simulink model "generalModelForErrorsNEW"  (R2016b)
settings: Solver=ode15s  StartTime=0  StopTime=3500  FixedStep=0.0001  MaxStep=0.001  RelTol=1e-3
values from neighbouring files (symbols this model uses):
  bigpump_const = 1    [run_model.m]
  gain_coef = 4000*10    (= 40000)    [params.m]    (also in run_model.m)
  min_vol = 20    [params.m]
  minipump_const = 0    [run_model.m]
  pipe_diameter = 2    [params.m]
  pressurization = 100000    [params.m]
  pump_speed = 20000    [params.m]
  valve_gain = 0.01    [params.m]
  ws_fault_time = fault_time    [run_model.m]
  ws_sample_time_end_valve_bigpump_in = 0    [run_model.m]
  ws_sample_time_end_valve_bigpump_out = 0    [run_model.m]
  ws_sample_time_end_valve_car_tank = 0    [run_model.m]
  ws_sample_time_end_valve_cartank1_in = 0    [run_model.m]
  ws_sample_time_end_valve_cartank1_out = 0    [run_model.m]
  ws_sample_time_end_valve_cartank2_in = 0    [run_model.m]
  ws_sample_time_end_valve_cartank2_out = 0    [run_model.m]
  ws_sample_time_end_valve_cartank3_in = 0    [run_model.m]
  ws_sample_time_end_valve_cartank3_out = 0    [run_model.m]
  ws_sample_time_end_valve_general_tank = 0    [run_model.m]
  ws_sample_time_end_valve_minipump_in = 0    [run_model.m]
  ws_sample_time_end_valve_minipump_out = 0    [run_model.m]
undefined symbols (not defined in the file or in its folder): sigbuilder_block
libraries: sh_lib x61, nesl_utility x34, fl_lib x32, powerlib_meascontrol x2
(part 1 of 2)
settings Model: Creator=plotb  LastModifiedBy=plotb
settings SimscapeCC: SimscapeLogDataHistory=10000

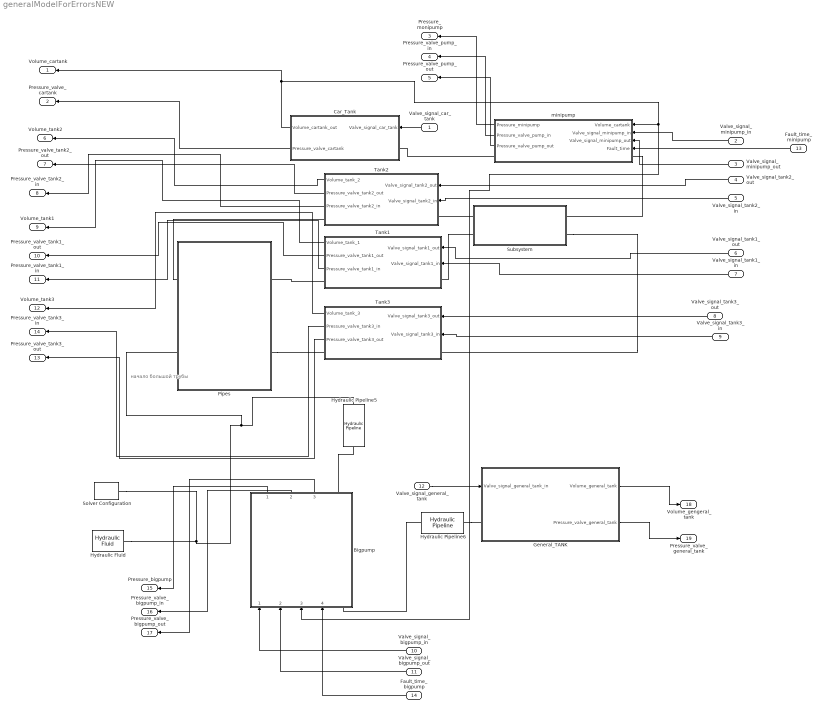
== system generalModelForErrorsNEW ==
  note: начало большой трубы
  Valve_signal_car_tank : Inport
  Valve_signal_minipump_in : Inport  Port=2
  Valve_signal_minipump_out : Inport  Port=3
  Valve_signal_tank2_out : Inport  Port=4
  Valve_signal_tank2_in : Inport  Port=5
  Valve_signal_tank1_out : Inport  Port=6
  Valve_signal_tank1_in : Inport  Port=7
  Valve_signal_tank3_out : Inport  Port=8
  Valve_signal_tank3_in : Inport  Port=9
  Valve_signal_bigpump_in : Inport  Port=10
  Valve_signal_bigpump_out : Inport  Port=11
  Valve_signal_general_tank : Inport  Port=12
  Fault_time_minipump : Inport  Port=13
  Fault_time_bigpump : Inport  Port=14
  Bigpump : Subsystem
  Car_Tank : Subsystem
  General_TANK : Subsystem
  Hydraulic Fluid : sh_lib/Hydraulic Utilities/Hydraulic Fluid  DataSource=1  SelFluid=21  SysTemp=temp  TrapAir=0.005  ViscDerFactor=1  range_error=1
  Hydraulic Pipeline5 : sh_lib/Pipelines/Hydraulic Pipeline  cs_type=1  d_in=pipe_diameter*2 m  area=1e-4 m^2  D_h=0.0112 m  s_factor=64  length=pipe_length_long m  length_ad=1 m  roughness=1.5e-5 m  Re_lam=2e+3  Re_turb=4e+3  wall_type=1  pr_r_coef=2e-12 m/Pa  time_const=0.01 s  k_sh=1.4  initial_pressure=initial_pressure Pa
  Hydraulic Pipeline6 : sh_lib/Pipelines/Hydraulic Pipeline  cs_type=1  d_in=pipe_diameter*2 m  area=1e-4 m^2  D_h=0.0112 m  s_factor=64  length=pipe_length_long m  length_ad=1 m  roughness=1.5e-5 m  Re_lam=2e+3  Re_turb=4e+3  wall_type=1  pr_r_coef=2e-12 m/Pa  time_const=0.01 s  k_sh=1.4  initial_pressure=initial_pressure Pa
  Pipes : Subsystem
  Solver Configuration : nesl_utility/Solver Configuration  PhysicalDomain=network_engine_domain  SubClassName=solver  LeftPortType=input  RightPortType=generic  Accelerate=off  Tones=[]  Harmonics=[]  SimulateNoise=off  Profile=off  UseLocalSampling=off  EnableSwitchedLinearOptims=on  FrequencyDomain=off  UseCCode=off  RelTol=0.001  AbsTol=1e-06  MinStep=1e-09  ToWorkspace=off  RevertToSquareIcSolve=off  NumHomotopyIterations=100  PhasorMode=off  PhasorModeNumHarmonics=1  OverrideAbsTol=off  DoDC=off  ResidualTolerance=1e-09  UseLocalSolver=off  LocalSolverChoice=NE_BACKWARD_EULER_ADVANCER  LocalSolverSampleTime=0.001  DoFixedCost=off  MaxNonlinIter=3  MaxModeIter=2  LinearAlgebra=Sparse  DelaysMemoryBudget=1024  AutomaticFiltering=on  FilteringTimeConstant=0.001
  Subsystem : Subsystem
  Tank1 : Subsystem
  Tank2 : Subsystem
  Tank3 : Subsystem
  minipump : Subsystem
  Volume_cartank : Outport
  Pressure_valve_cartank : Outport  Port=2
  Pressure_monipump : Outport  Port=3
  Pressure_valve_pump_in : Outport  Port=4
  Pressure_valve_pump_out : Outport  Port=5
  Volume_tank2 : Outport  Port=6
  Pressure_valve_tank2_out : Outport  Port=7
  Pressure_valve_tank2_in : Outport  Port=8
  Volume_tank1 : Outport  Port=9
  Pressure_valve_tank1_out : Outport  Port=10
  Pressure_valve_tank1_in : Outport  Port=11
  Volume_tank3 : Outport  Port=12
  Pressure_valve_tank3_out : Outport  Port=13
  Pressure_valve_tank3_in : Outport  Port=14
  Pressure_bigpump : Outport  Port=15
  Pressure_valve_bigpump_in : Outport  Port=16
  Pressure_valve_bigpump_out : Outport  Port=17
  Volume_gengeral_tank : Outport  Port=18
  Pressure_valve_general_tank : Outport  Port=19
  wires:
  Tank2/1(Volume_tank_2) -> Volume_tank2/1
  General_TANK/1(Volume_general_tank) -> Volume_gengeral_tank/1
  Tank1/1(Volume_tank_1) -> Volume_tank1/1
  Tank3/1(Volume_tank_3) -> Volume_tank3/1
  Valve_signal_car_tank/1 -> Car_Tank/1(Valve_signal_car_tank)
  Valve_signal_minipump_in/1 -> minipump/2(Valve_signal_minipump_in)
  Valve_signal_minipump_out/1 -> minipump/3(Valve_signal_minipump_out)
  Valve_signal_tank2_out/1 -> Tank2/1(Valve_signal_tank2_out)
  Valve_signal_tank2_in/1 -> Tank2/2(Valve_signal_tank2_in)
  Valve_signal_tank1_out/1 -> Tank1/1(Valve_signal_tank1_out)
  Valve_signal_tank1_in/1 -> Tank1/2(Valve_signal_tank1_in)
  Valve_signal_tank3_out/1 -> Tank3/1(Valve_signal_tank3_out)
  Valve_signal_tank3_in/1 -> Tank3/2(Valve_signal_tank3_in)
  Valve_signal_bigpump_in/1 -> Bigpump/1(Valve_signal_bigpump_in)
  Valve_signal_bigpump_out/1 -> Bigpump/2(Valve_signal_bigpump_out)
  Valve_signal_general_tank/1 -> General_TANK/1(Valve_signal_general_tank_in)
  Car_Tank/2(Pressure_valve_cartank) -> Pressure_valve_cartank/1
  Car_Tank/1(Volume_cartank_out) -> Bigpump/3(Volume_cartank), minipump/1(Volume_cartank), Volume_cartank/1
  Fault_time_minipump/1 -> minipump/4(Fault_time)
  minipump/1(Pressure_minipump) -> Pressure_monipump/1
  minipump/2(Pressure_valve_pump_in) -> Pressure_valve_pump_in/1
  minipump/3(Pressure_valve_pump_out) -> Pressure_valve_pump_out/1
  Tank2/2(Pressure_valve_tank2_out) -> Pressure_valve_tank2_out/1
  Tank2/3(Pressure_valve_tank2_in) -> Pressure_valve_tank2_in/1
  Tank1/2(Pressure_valve_tank1_out) -> Pressure_valve_tank1_out/1
  Tank1/3(Pressure_valve_tank1_in) -> Pressure_valve_tank1_in/1
  Tank3/2(Pressure_valve_tank3_in) -> Pressure_valve_tank3_in/1
  Tank3/3(Pressure_valve_tank3_out) -> Pressure_valve_tank3_out/1
  Fault_time_bigpump/1 -> Bigpump/4(Fault_time_bigpump)
  Bigpump/1(Pressure_bigpump) -> Pressure_bigpump/1
  Bigpump/2(Pressure_valve_bigpump_in) -> Pressure_valve_bigpump_in/1
  Bigpump/3(Pressure_valve_bigpump_out) -> Pressure_valve_bigpump_out/1
  General_TANK/2(Pressure_valve_general_tank) -> Pressure_valve_general_tank/1
  connections:
  minipump/LConn1 -- Subsystem/RConn1
  Subsystem/LConn1 -- Tank2/LConn1
  Subsystem/LConn2 -- Tank1/LConn1
  Hydraulic Fluid/RConn1 -- Pipes/LConn2 -- Hydraulic Pipeline5/LConn1 -- Solver Configuration/RConn1
  Tank2/RConn1 -- Pipes/LConn1
  Tank1/RConn1 -- Pipes/RConn1
  Pipes/RConn2 -- Tank3/RConn1
  Hydraulic Pipeline6/RConn1 -- General_TANK/LConn1
  Hydraulic Pipeline6/LConn1 -- Bigpump/LConn1
  Hydraulic Pipeline5/RConn1 -- Bigpump/RConn1
  minipump/RConn1 -- Car_Tank/LConn1
  Subsystem/RConn2 -- Tank3/LConn1

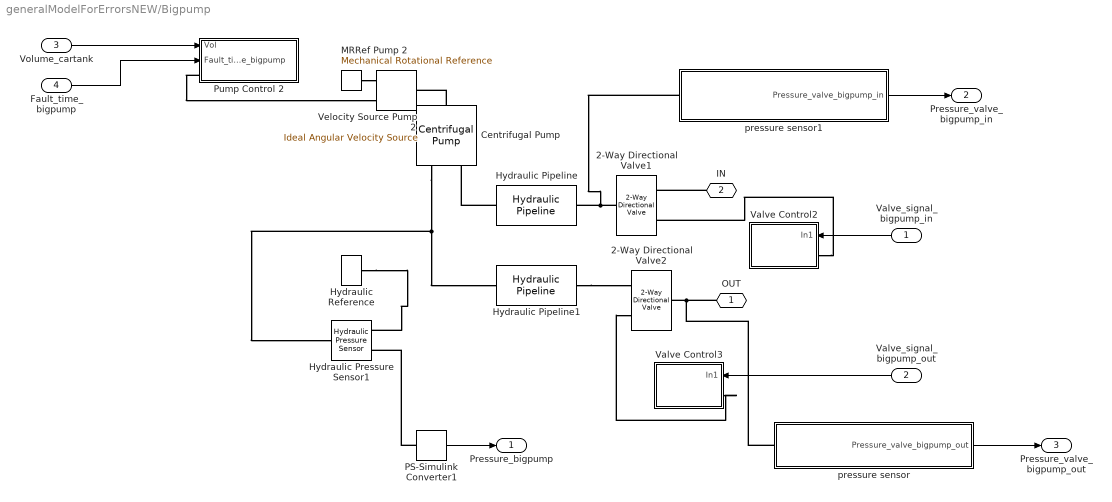
== system generalModelForErrorsNEW/Bigpump ==
  Valve_signal_bigpump_in : Inport
  Valve_signal_bigpump_out : Inport  Port=2
  Volume_cartank : Inport  Port=3
  Fault_time_bigpump : Inport  Port=4
  2-Way Directional Valve1 : sh_lib/Valves/Directional Valves/2-Way Directional Valve  mdl_type=1  area_max=passage_max_area_big_pipe m^2  opening_max=valve_stroke m  opening_tab=[ -0.002 0 0.002 0.005 0.015 ] m  area_tab=[ 1e-9 2.0352e-7 4.0736e-5 1.1438e-4 3.4356e-4 ] m^2  pressure_tab=[ -1e+7 -5e+6 -2e+6 2e+6 5e+6 1e+7 ] Pa  flow_rate_tab=[ -1e-7 -7.0711e-8 -4.4721e-8 4.4721e-8 7.0711e-8 1e-7; -2.0352e-5 -1.4391e-5 -9.1017e-6 9.1017e-6 1.4391e-5 2.0352e-5; -0.0040736 -0.0028805 -0.0018218 0.0018218 0.0028805 0.0040736; -0.011438 -0.0080879 -0.0051152 0.0051152 0.0080879 0.011438; -0.034356 -0.024293 -0.015364 0.015364 0.024293 0.034356 ] m^3/s  interp_method=1  extrap_method=1  C_d=0.7  x_0=valve_stroke m  Re_cr=12  A_leak=1e-12 m^2
  2-Way Directional Valve2 : sh_lib/Valves/Directional Valves/2-Way Directional Valve  mdl_type=1  area_max=passage_max_area_big_pipe m^2  opening_max=valve_stroke m  opening_tab=[ -0.002 0 0.002 0.005 0.015 ] m  area_tab=[ 1e-9 2.0352e-7 4.0736e-5 1.1438e-4 3.4356e-4 ] m^2  pressure_tab=[ -1e+7 -5e+6 -2e+6 2e+6 5e+6 1e+7 ] Pa  flow_rate_tab=[ -1e-7 -7.0711e-8 -4.4721e-8 4.4721e-8 7.0711e-8 1e-7; -2.0352e-5 -1.4391e-5 -9.1017e-6 9.1017e-6 1.4391e-5 2.0352e-5; -0.0040736 -0.0028805 -0.0018218 0.0018218 0.0028805 0.0040736; -0.011438 -0.0080879 -0.0051152 0.0051152 0.0080879 0.011438; -0.034356 -0.024293 -0.015364 0.015364 0.024293 0.034356 ] m^3/s  interp_method=1  extrap_method=1  C_d=0.7  x_0=valve_stroke m  Re_cr=12  A_leak=1e-12 m^2
  Centrifugal Pump : sh_lib/Pumps and Motors/Centrifugal Pump  mdl_type=1  c_1=326.8 Pa/(kg/m^3)  c_2=3.104e+4 Pa*s/kg  c_3=1.097e+7 Pa*s^2/(kg*m^3)  c_4=2.136e+5 Pa*s^2/(kg*m^3)  c_f=0.8  design_del=130 lpm  ref_velocity=1.77e+3 rpm  ref_density=920 kg/m^3  leak_resistance=1e+8 Pa/(m^3/s)  T_const=0.1 N*m  trq_press_coeff=1e-6 N*m/Pa  pump_del_1D=[ 0 28 90 130 154 182 ] lpm  press_diff_1D=[ 2.6 2.4 2 1.6 1.2 0.8 ] bar  pump_del_power_1D=[ 0 20 40 60 80 100 120 140 160 ] lpm  power_1D=[ 220 280 310 360 390 420 480 500 550 ] W  pump_del_2D=[ 0 50 100 150 200 250 300 350 ] lpm  pump_vel_2D=[ 3.2e+3 3.3e+3 3.4e+3 3.5e+3 ] rpm  press_diff_2D=[ 8.300000000000001 8.800000000000001 9.300000000000001 9.9; 7.8 8.300000000000001 8.800000000000001 9.4; 7.2 7.6 8.199999999999999 8.699999999999999; 6.5 7 7.5 8; 5.6 6.1 6.6 7.1; 4.7 5.2 5.7 6.2; 3.4 4 4.4 4.9; 2.3 2.7 3.4 3.6 ] bar  pump_del_power_2D=[ 0 50 100 150 200 250 300 350 ] lpm  power_2D=[ 1.223e+3 1.341e+3 1.467e+3 1.6e+3; 1.414e+3 1.551e+3 1.696e+3 1.85e+3; 1.636e+3 1.794e+3 1.962e+3 2.14e+3; 1.941e+3 2.129e+3 2.326e+3 2.54e+3; 2.224e+3 2.439e+3 2.66e+3 2.91e+3; 2.453e+3 2.691e+3 2.947e+3 3.21e+3; 2.757e+3 3.024e+3 3.307e+3 3.608e+3; 2.945e+3 3.23e+3 3.533e+3 3.854e+3 ] W  interp_method=1  extrap_method=1
  Hydraulic Pipeline : sh_lib/Pipelines/Hydraulic Pipeline  cs_type=1  d_in=pipe_diameter*2 m  area=1e-4 m^2  D_h=0.0112 m  s_factor=64  length=pipe_length_short m  length_ad=1 m  roughness=1.5e-5 m  Re_lam=2e+3  Re_turb=4e+3  wall_type=1  pr_r_coef=2e-12 m/Pa  time_const=0.01 s  k_sh=1.4  initial_pressure=initial_pressure Pa
  Hydraulic Pipeline1 : sh_lib/Pipelines/Hydraulic Pipeline  cs_type=1  d_in=pipe_diameter*2 m  area=1e-4 m^2  D_h=0.0112 m  s_factor=64  length=pipe_length_short m  length_ad=1 m  roughness=1.5e-5 m  Re_lam=2e+3  Re_turb=4e+3  wall_type=1  pr_r_coef=2e-12 m/Pa  time_const=0.01 s  k_sh=1.4  initial_pressure=initial_pressure Pa
  Hydraulic Pressure Sensor1 : fl_lib/Hydraulic/Hydraulic Sensors/Hydraulic Pressure Sensor
  Hydraulic Reference : fl_lib/Hydraulic/Hydraulic Elements/Hydraulic Reference
  MRRef Pump 2 : fl_lib/Mechanical/Rotational Elements/Mechanical Rotational Reference
  PS-Simulink Converter1 : nesl_utility/PS-Simulink Converter  PhysicalDomain=network_engine_domain  SubClassName=ps_output  LeftPortType=input  RightPortType=output  PseudoPeriodic=off  Frequencies=[]  Unit=1  AffineConversion=off
  Pump Control 2 : Subsystem
  Valve Control2 : Subsystem
  Valve Control3 : Subsystem
  Velocity Source Pump 2 : fl_lib/Mechanical/Mechanical Sources/Ideal Angular Velocity Source
  pressure sensor : Subsystem
  pressure sensor1 : Subsystem
  OUT : PMIOPort  Port=1  Side=Left
  IN : PMIOPort  Port=2  Side=Right
  Pressure_bigpump : Outport
  Pressure_valve_bigpump_in : Outport  Port=2
  Pressure_valve_bigpump_out : Outport  Port=3
  wires:
  PS-Simulink Converter1/1 -> Pressure_bigpump/1
  Valve_signal_bigpump_out/1 -> Valve Control3/1(In1)
  Valve_signal_bigpump_in/1 -> Valve Control2/1(In1)
  Volume_cartank/1 -> Pump Control 2/1(Vol)
  Fault_time_bigpump/1 -> Pump Control 2/2(Fault_time_bigpump)
  pressure sensor1/1(Pressure_valve_bigpump_in) -> Pressure_valve_bigpump_in/1
  pressure sensor/1(Pressure_valve_bigpump_out) -> Pressure_valve_bigpump_out/1
  connections:
  2-Way Directional Valve1/RConn1 -- pressure sensor1/LConn1 -- Hydraulic Pipeline/LConn1
  Hydraulic Pipeline/RConn1 -- Centrifugal Pump/RConn2
  Hydraulic Pipeline1/RConn1 -- 2-Way Directional Valve2/LConn2
  OUT/RConn1 -- pressure sensor/LConn1 -- 2-Way Directional Valve2/RConn1
  MRRef Pump 2/LConn1 -- Velocity Source Pump 2/RConn2
  Centrifugal Pump/LConn1 -- Velocity Source Pump 2/LConn1
  PS-Simulink Converter1/LConn1 -- Hydraulic Pressure Sensor1/RConn2
  IN/RConn1 -- 2-Way Directional Valve1/LConn2
  Pump Control 2/LConn1 -- Velocity Source Pump 2/RConn1
  Centrifugal Pump/RConn1 -- Hydraulic Pressure Sensor1/LConn1 -- Hydraulic Pipeline1/LConn1
  Hydraulic Reference/LConn1 -- Hydraulic Pressure Sensor1/RConn1
  Valve Control2/LConn1 -- 2-Way Directional Valve1/LConn1
  Valve Control3/LConn1 -- 2-Way Directional Valve2/LConn1

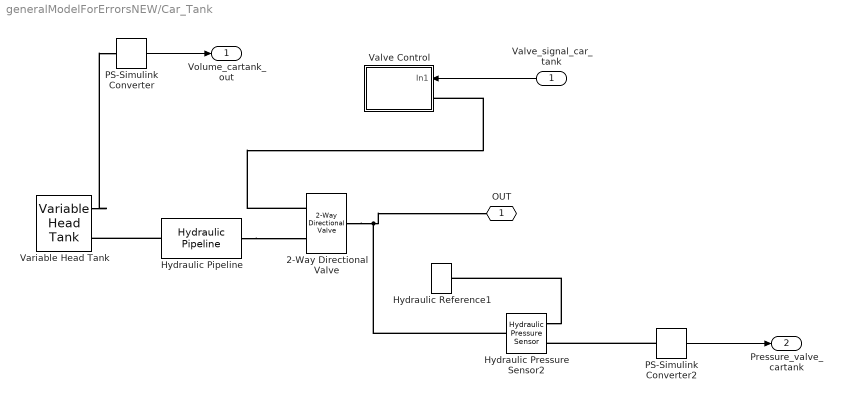
== system generalModelForErrorsNEW/Car_Tank ==
  Valve_signal_car_tank : Inport
  2-Way Directional Valve : sh_lib/Valves/Directional Valves/2-Way Directional Valve  mdl_type=1  area_max=passage_max_area m^2  opening_max=valve_stroke m  opening_tab=[ -0.002 0 0.002 0.005 0.015 ] m  area_tab=[ 1e-9 2.0352e-7 4.0736e-5 1.1438e-4 3.4356e-4 ] m^2  pressure_tab=[ -1e+7 -5e+6 -2e+6 2e+6 5e+6 1e+7 ] Pa  flow_rate_tab=[ -1e-7 -7.0711e-8 -4.4721e-8 4.4721e-8 7.0711e-8 1e-7; -2.0352e-5 -1.4391e-5 -9.1017e-6 9.1017e-6 1.4391e-5 2.0352e-5; -0.0040736 -0.0028805 -0.0018218 0.0018218 0.0028805 0.0040736; -0.011438 -0.0080879 -0.0051152 0.0051152 0.0080879 0.011438; -0.034356 -0.024293 -0.015364 0.015364 0.024293 0.034356 ] m^3/s  interp_method=1  extrap_method=1  C_d=0.7  x_0=valve_stroke m  Re_cr=12  A_leak=1e-12 m^2
  Hydraulic Pipeline : sh_lib/Pipelines/Hydraulic Pipeline  cs_type=1  d_in=pipe_diameter m  area=1e-4 m^2  D_h=0.0112 m  s_factor=64  length=pipe_length_short m  length_ad=1 m  roughness=1.5e-5 m  Re_lam=2e+3  Re_turb=4e+3  wall_type=1  pr_r_coef=2e-12 m/Pa  time_const=0.01 s  k_sh=1.4  initial_pressure=initial_pressure Pa
  Hydraulic Pressure Sensor2 : fl_lib/Hydraulic/Hydraulic Sensors/Hydraulic Pressure Sensor
  Hydraulic Reference1 : fl_lib/Hydraulic/Hydraulic Elements/Hydraulic Reference
  PS-Simulink Converter : nesl_utility/PS-Simulink Converter  PhysicalDomain=network_engine_domain  SubClassName=ps_output  LeftPortType=input  RightPortType=output  PseudoPeriodic=off  Frequencies=[]  Unit=1  AffineConversion=off
  PS-Simulink Converter2 : nesl_utility/PS-Simulink Converter  PhysicalDomain=network_engine_domain  SubClassName=ps_output  LeftPortType=input  RightPortType=output  PseudoPeriodic=off  Frequencies=[]  Unit=1  AffineConversion=off
  Valve Control : Subsystem
  Variable Head Tank : sh_lib/Low-Pressure Blocks/Variable Head Tank  init_volume=initial_fluid_volume m^3  press=pressurization/2 Pa  level_spec=1  tank_area=tank_cross_section_area_big m^2  fluid_volume_tab=[ 0 0.0028 0.0065 0.0114 0.0176 0.0252 0.0344 0.0436 0.0512 0.0574 0.0623 0.066 0.0688 0.0707 0.07199999999999999 0.0727 ] m^3  fluid_level_tab=[ 0 0.02 0.04 0.06 0.08 0.1 0.12 0.14 0.16 0.18 0.2 0.22 0.24 0.26 0.28 0.3 ] m  pipe_diam=pipe_diameter m  loss_coeff=1.2  interp_method=1  extrap_method=1
  OUT : PMIOPort  Port=1  Side=Left
  Volume_cartank_out : Outport
  Pressure_valve_cartank : Outport  Port=2
  wires:
  PS-Simulink Converter/1 -> Volume_cartank_out/1
  PS-Simulink Converter2/1 -> Pressure_valve_cartank/1
  Valve_signal_car_tank/1 -> Valve Control/1(In1)
  connections:
  Hydraulic Pipeline/LConn1 -- Variable Head Tank/RConn2
  Variable Head Tank/RConn1 -- PS-Simulink Converter/LConn1
  Hydraulic Pipeline/RConn1 -- 2-Way Directional Valve/LConn2
  2-Way Directional Valve/RConn1 -- Hydraulic Pressure Sensor2/LConn1 -- OUT/RConn1
  PS-Simulink Converter2/LConn1 -- Hydraulic Pressure Sensor2/RConn2
  2-Way Directional Valve/LConn1 -- Valve Control/LConn1
  Hydraulic Pressure Sensor2/RConn1 -- Hydraulic Reference1/LConn1

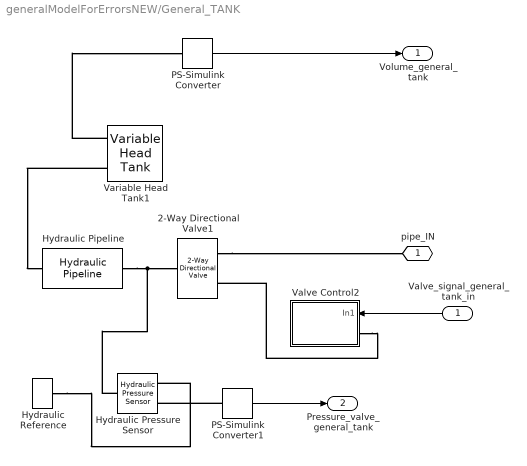
== system generalModelForErrorsNEW/General_TANK ==
  Valve_signal_general_tank_in : Inport
  2-Way Directional Valve1 : sh_lib/Valves/Directional Valves/2-Way Directional Valve  mdl_type=1  area_max=passage_max_area_big_pipe m^2  opening_max=valve_stroke m  opening_tab=[ -0.002 0 0.002 0.005 0.015 ] m  area_tab=[ 1e-9 2.0352e-7 4.0736e-5 1.1438e-4 3.4356e-4 ] m^2  pressure_tab=[ -1e+7 -5e+6 -2e+6 2e+6 5e+6 1e+7 ] Pa  flow_rate_tab=[ -1e-7 -7.0711e-8 -4.4721e-8 4.4721e-8 7.0711e-8 1e-7; -2.0352e-5 -1.4391e-5 -9.1017e-6 9.1017e-6 1.4391e-5 2.0352e-5; -0.0040736 -0.0028805 -0.0018218 0.0018218 0.0028805 0.0040736; -0.011438 -0.0080879 -0.0051152 0.0051152 0.0080879 0.011438; -0.034356 -0.024293 -0.015364 0.015364 0.024293 0.034356 ] m^3/s  interp_method=1  extrap_method=1  C_d=0.7  x_0=valve_stroke m  Re_cr=12  A_leak=1e-12 m^2
  Hydraulic Pipeline : sh_lib/Pipelines/Hydraulic Pipeline  cs_type=1  d_in=pipe_diameter*2 m  area=1e-4 m^2  D_h=0.0112 m  s_factor=64  length=pipe_length_short m  length_ad=1 m  roughness=1.5e-5 m  Re_lam=2e+3  Re_turb=4e+3  wall_type=1  pr_r_coef=2e-12 m/Pa  time_const=0.01 s  k_sh=1.4  initial_pressure=initial_pressure Pa
  Hydraulic Pressure Sensor : fl_lib/Hydraulic/Hydraulic Sensors/Hydraulic Pressure Sensor
  Hydraulic Reference : fl_lib/Hydraulic/Hydraulic Elements/Hydraulic Reference
  PS-Simulink Converter : nesl_utility/PS-Simulink Converter  PhysicalDomain=network_engine_domain  SubClassName=ps_output  LeftPortType=input  RightPortType=output  PseudoPeriodic=off  Frequencies=[]  Unit=1  AffineConversion=off
  PS-Simulink Converter1 : nesl_utility/PS-Simulink Converter  PhysicalDomain=network_engine_domain  SubClassName=ps_output  LeftPortType=input  RightPortType=output  PseudoPeriodic=off  Frequencies=[]  Unit=1  AffineConversion=off
  Valve Control2 : Subsystem
  Variable Head Tank1 : sh_lib/Low-Pressure Blocks/Variable Head Tank  init_volume=10 m^3  press=0 Pa  level_spec=1  tank_area=50 m^2  fluid_volume_tab=[ 0 0.0028 0.0065 0.0114 0.0176 0.0252 0.0344 0.0436 0.0512 0.0574 0.0623 0.066 0.0688 0.0707 0.07199999999999999 0.0727 ] m^3  fluid_level_tab=[ 0 0.02 0.04 0.06 0.08 0.1 0.12 0.14 0.16 0.18 0.2 0.22 0.24 0.26 0.28 0.3 ] m  pipe_diam=5 m  loss_coeff=1.2  interp_method=1  extrap_method=1
  pipe_IN : PMIOPort  Port=1  Side=Left
  Volume_general_tank : Outport
  Pressure_valve_general_tank : Outport  Port=2
  wires:
  PS-Simulink Converter/1 -> Volume_general_tank/1
  Valve_signal_general_tank_in/1 -> Valve Control2/1(In1)
  PS-Simulink Converter1/1 -> Pressure_valve_general_tank/1
  connections:
  Variable Head Tank1/RConn2 -- Hydraulic Pipeline/RConn1
  Hydraulic Pipeline/LConn1 -- Hydraulic Pressure Sensor/LConn1 -- 2-Way Directional Valve1/RConn1
  2-Way Directional Valve1/LConn2 -- pipe_IN/RConn1
  Variable Head Tank1/RConn1 -- PS-Simulink Converter/LConn1
  Valve Control2/LConn1 -- 2-Way Directional Valve1/LConn1
  PS-Simulink Converter1/LConn1 -- Hydraulic Pressure Sensor/RConn2
  Hydraulic Reference/LConn1 -- Hydraulic Pressure Sensor/RConn1

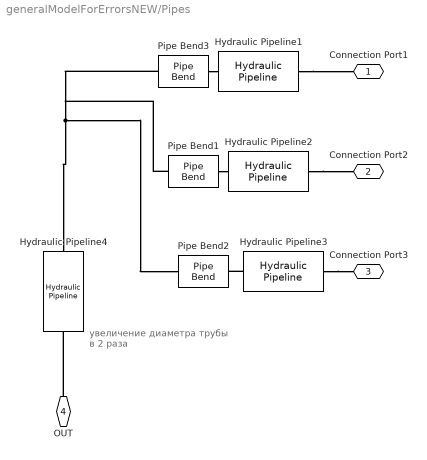
== system generalModelForErrorsNEW/Pipes ==
  note: увеличение диаметра трубы в 2 раза
  Hydraulic Pipeline1 : sh_lib/Pipelines/Hydraulic Pipeline  cs_type=1  d_in=pipe_diameter m  area=1e-4 m^2  D_h=0.0112 m  s_factor=64  length=pipe_length_long m  length_ad=1 m  roughness=1.5e-5 m  Re_lam=2e+3  Re_turb=4e+3  wall_type=1  pr_r_coef=2e-12 m/Pa  time_const=0.01 s  k_sh=1.4  initial_pressure=initial_pressure Pa
  Hydraulic Pipeline2 : sh_lib/Pipelines/Hydraulic Pipeline  cs_type=1  d_in=pipe_diameter m  area=1e-4 m^2  D_h=0.0112 m  s_factor=64  length=pipe_length_long m  length_ad=1 m  roughness=1.5e-5 m  Re_lam=2e+3  Re_turb=4e+3  wall_type=1  pr_r_coef=2e-12 m/Pa  time_const=0.01 s  k_sh=1.4  initial_pressure=initial_pressure Pa
  Hydraulic Pipeline3 : sh_lib/Pipelines/Hydraulic Pipeline  cs_type=1  d_in=pipe_diameter m  area=1e-4 m^2  D_h=0.0112 m  s_factor=64  length=pipe_length_long m  length_ad=1 m  roughness=1.5e-5 m  Re_lam=2e+3  Re_turb=4e+3  wall_type=1  pr_r_coef=2e-12 m/Pa  time_const=0.01 s  k_sh=1.4  initial_pressure=initial_pressure Pa
  Hydraulic Pipeline4 : sh_lib/Pipelines/Hydraulic Pipeline  cs_type=1  d_in=pipe_diameter*2 m  area=1e-4 m^2  D_h=0.0112 m  s_factor=64  length=pipe_length_long m  length_ad=1 m  roughness=1.5e-5 m  Re_lam=2e+3  Re_turb=4e+3  wall_type=1  pr_r_coef=2e-12 m/Pa  time_const=0.01 s  k_sh=1.4  initial_pressure=initial_pressure Pa
  Pipe Bend1 : sh_lib/Local Hydraulic Resistances/Pipe Bend  pipe_diam=pipe_diameter m  bend_rad=5 m  bend_angle=90 deg  roughness=1.5e-5 m  Re_cr=350
  Pipe Bend2 : sh_lib/Local Hydraulic Resistances/Pipe Bend  pipe_diam=pipe_diameter m  bend_rad=5 m  bend_angle=90 deg  roughness=1.5e-5 m  Re_cr=350
  Pipe Bend3 : sh_lib/Local Hydraulic Resistances/Pipe Bend  pipe_diam=pipe_diameter m  bend_rad=5 m  bend_angle=90 deg  roughness=1.5e-5 m  Re_cr=350
  Connection Port1 : PMIOPort  Port=1  Side=Right
  Connection Port2 : PMIOPort  Port=2  Side=Left
  Connection Port3 : PMIOPort  Port=3  Side=Right
  OUT : PMIOPort  Port=4  Side=Left
  connections:
  Hydraulic Pipeline1/LConn1 -- Connection Port1/RConn1
  Hydraulic Pipeline2/LConn1 -- Connection Port2/RConn1
  Hydraulic Pipeline3/LConn1 -- Connection Port3/RConn1
  Hydraulic Pipeline3/RConn1 -- Pipe Bend2/LConn1
  Pipe Bend1/LConn1 -- Hydraulic Pipeline2/RConn1
  Pipe Bend3/LConn1 -- Hydraulic Pipeline1/RConn1
  Pipe Bend3/RConn1 -- Pipe Bend1/RConn1 -- Pipe Bend2/RConn1 -- Hydraulic Pipeline4/LConn1
  OUT/RConn1 -- Hydraulic Pipeline4/RConn1

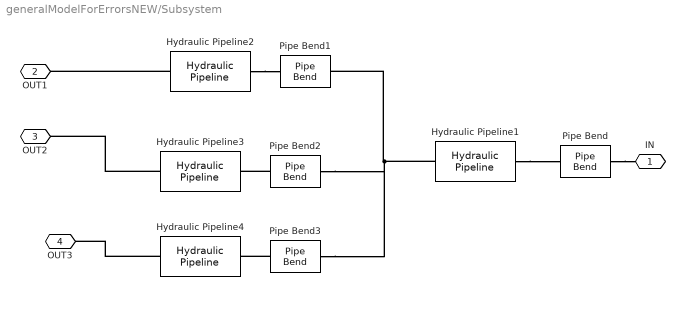
== system generalModelForErrorsNEW/Subsystem ==
  Hydraulic Pipeline{1..4} (4 alike) : sh_lib/Pipelines/Hydraulic Pipeline  cs_type=1  d_in=pipe_diameter m  area=1e-4 m^2  D_h=0.0112 m  s_factor=64  length=pipe_length_short m  length_ad=1 m  roughness=1.5e-5 m  Re_lam=2e+3  Re_turb=4e+3  wall_type=1  pr_r_coef=2e-12 m/Pa  time_const=0.01 s  k_sh=1.4  initial_pressure=initial_pressure Pa
  Pipe Bend{,1..3} (4 alike) : sh_lib/Local Hydraulic Resistances/Pipe Bend  pipe_diam=pipe_diameter m  bend_rad=5 m  bend_angle=90 deg  roughness=1.5e-5 m  Re_cr=350
  IN : PMIOPort  Port=1  Side=Right
  OUT1 : PMIOPort  Port=2  Side=Left
  OUT2 : PMIOPort  Port=3  Side=Left
  OUT3 : PMIOPort  Port=4  Side=Right
  connections:
  Pipe Bend/LConn1 -- IN/RConn1
  Hydraulic Pipeline1/LConn1 -- Pipe Bend/RConn1
  Pipe Bend2/RConn1 -- Hydraulic Pipeline3/LConn1
  Pipe Bend3/RConn1 -- Hydraulic Pipeline4/LConn1
  Hydraulic Pipeline2/LConn1 -- Pipe Bend1/RConn1
  Hydraulic Pipeline1/RConn1 -- Pipe Bend3/LConn1 -- Pipe Bend2/LConn1 -- Pipe Bend1/LConn1
  Hydraulic Pipeline2/RConn1 -- OUT1/RConn1
  Hydraulic Pipeline3/RConn1 -- OUT2/RConn1
  Hydraulic Pipeline4/RConn1 -- OUT3/RConn1

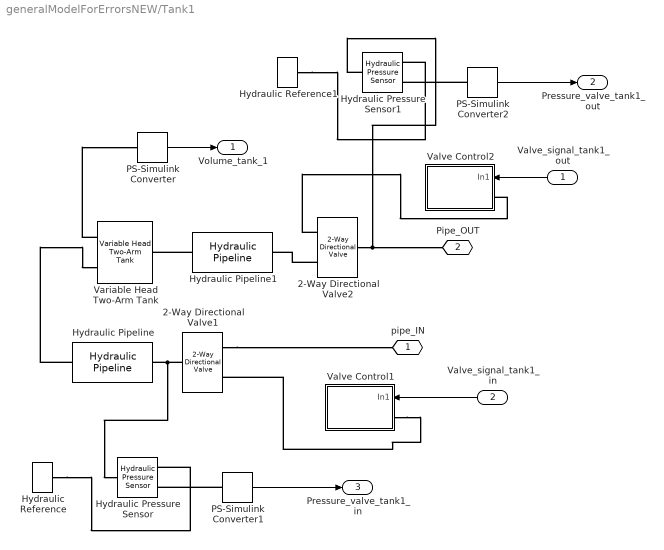
== system generalModelForErrorsNEW/Tank1 ==
  Valve_signal_tank1_out : Inport
  Valve_signal_tank1_in : Inport  Port=2
  2-Way Directional Valve1 : sh_lib/Valves/Directional Valves/2-Way Directional Valve  mdl_type=1  area_max=passage_max_area m^2  opening_max=valve_stroke m  opening_tab=[ -0.002 0 0.002 0.005 0.015 ] m  area_tab=[ 1e-9 2.0352e-7 4.0736e-5 1.1438e-4 3.4356e-4 ] m^2  pressure_tab=[ -1e+7 -5e+6 -2e+6 2e+6 5e+6 1e+7 ] Pa  flow_rate_tab=[ -1e-7 -7.0711e-8 -4.4721e-8 4.4721e-8 7.0711e-8 1e-7; -2.0352e-5 -1.4391e-5 -9.1017e-6 9.1017e-6 1.4391e-5 2.0352e-5; -0.0040736 -0.0028805 -0.0018218 0.0018218 0.0028805 0.0040736; -0.011438 -0.0080879 -0.0051152 0.0051152 0.0080879 0.011438; -0.034356 -0.024293 -0.015364 0.015364 0.024293 0.034356 ] m^3/s  interp_method=1  extrap_method=1  C_d=0.7  x_0=valve_stroke m  Re_cr=12  A_leak=1e-12 m^2
  2-Way Directional Valve2 : sh_lib/Valves/Directional Valves/2-Way Directional Valve  mdl_type=1  area_max=passage_max_area m^2  opening_max=valve_stroke m  opening_tab=[ -0.002 0 0.002 0.005 0.015 ] m  area_tab=[ 1e-9 2.0352e-7 4.0736e-5 1.1438e-4 3.4356e-4 ] m^2  pressure_tab=[ -1e+7 -5e+6 -2e+6 2e+6 5e+6 1e+7 ] Pa  flow_rate_tab=[ -1e-7 -7.0711e-8 -4.4721e-8 4.4721e-8 7.0711e-8 1e-7; -2.0352e-5 -1.4391e-5 -9.1017e-6 9.1017e-6 1.4391e-5 2.0352e-5; -0.0040736 -0.0028805 -0.0018218 0.0018218 0.0028805 0.0040736; -0.011438 -0.0080879 -0.0051152 0.0051152 0.0080879 0.011438; -0.034356 -0.024293 -0.015364 0.015364 0.024293 0.034356 ] m^3/s  interp_method=1  extrap_method=1  C_d=0.7  x_0=valve_stroke m  Re_cr=12  A_leak=1e-12 m^2
  Hydraulic Pipeline : sh_lib/Pipelines/Hydraulic Pipeline  cs_type=1  d_in=pipe_diameter m  area=1e-4 m^2  D_h=0.0112 m  s_factor=64  length=pipe_length_short m  length_ad=1 m  roughness=1.5e-5 m  Re_lam=2e+3  Re_turb=4e+3  wall_type=1  pr_r_coef=2e-12 m/Pa  time_const=0.01 s  k_sh=1.4  initial_pressure=initial_pressure Pa
  Hydraulic Pipeline1 : sh_lib/Pipelines/Hydraulic Pipeline  cs_type=1  d_in=pipe_diameter m  area=1e-4 m^2  D_h=0.0112 m  s_factor=64  length=pipe_length_short m  length_ad=1 m  roughness=1.5e-5 m  Re_lam=2e+3  Re_turb=4e+3  wall_type=1  pr_r_coef=2e-12 m/Pa  time_const=0.01 s  k_sh=1.4  initial_pressure=initial_pressure Pa
  Hydraulic Pressure Sensor : fl_lib/Hydraulic/Hydraulic Sensors/Hydraulic Pressure Sensor
  Hydraulic Pressure Sensor1 : fl_lib/Hydraulic/Hydraulic Sensors/Hydraulic Pressure Sensor
  Hydraulic Reference : fl_lib/Hydraulic/Hydraulic Elements/Hydraulic Reference
  Hydraulic Reference1 : fl_lib/Hydraulic/Hydraulic Elements/Hydraulic Reference
  PS-Simulink Converter : nesl_utility/PS-Simulink Converter  PhysicalDomain=network_engine_domain  SubClassName=ps_output  LeftPortType=input  RightPortType=output  PseudoPeriodic=off  Frequencies=[]  Unit=1  AffineConversion=off
  PS-Simulink Converter1 : nesl_utility/PS-Simulink Converter  PhysicalDomain=network_engine_domain  SubClassName=ps_output  LeftPortType=input  RightPortType=output  PseudoPeriodic=off  Frequencies=[]  Unit=1  AffineConversion=off
  PS-Simulink Converter2 : nesl_utility/PS-Simulink Converter  PhysicalDomain=network_engine_domain  SubClassName=ps_output  LeftPortType=input  RightPortType=output  PseudoPeriodic=off  Frequencies=[]  Unit=1  AffineConversion=off
  Valve Control1 : Subsystem
  Valve Control2 : Subsystem
  Variable Head Two-Arm Tank : sh_lib/Low-Pressure Blocks/Variable Head Two-Arm Tank  init_volume=1 m^3  press=pressurization_mini Pa  level_spec=1  tank_area=10 m^2  fluid_volume_tab=[ 0 0.0028 0.0065 0.0114 0.0176 0.0252 0.0344 0.0436 0.0512 0.0574 0.0623 0.066 0.0688 0.0707 0.07199999999999999 0.0727 ] m^3  fluid_level_tab=[ 0 0.02 0.04 0.06 0.08 0.1 0.12 0.14 0.16 0.18 0.2 0.22 0.24 0.26 0.28 0.3 ] m  pipe_diam_A=pipe_diameter m  loss_coeff_A=1.2  pipe_diam_B=pipe_diameter m  height_B=portb_height m  loss_coeff_B=1.2  interp_method=1  extrap_method=1
  pipe_IN : PMIOPort  Port=1  Side=Left
  Pipe_OUT : PMIOPort  Port=2  Side=Right
  Volume_tank_1 : Outport
  Pressure_valve_tank1_out : Outport  Port=2
  Pressure_valve_tank1_in : Outport  Port=3
  wires:
  PS-Simulink Converter/1 -> Volume_tank_1/1
  Valve_signal_tank1_out/1 -> Valve Control2/1(In1)
  Valve_signal_tank1_in/1 -> Valve Control1/1(In1)
  PS-Simulink Converter1/1 -> Pressure_valve_tank1_in/1
  PS-Simulink Converter2/1 -> Pressure_valve_tank1_out/1
  connections:
  Hydraulic Pipeline1/LConn1 -- Variable Head Two-Arm Tank/LConn1
  Variable Head Two-Arm Tank/RConn1 -- PS-Simulink Converter/LConn1
  2-Way Directional Valve2/RConn1 -- Hydraulic Pressure Sensor1/LConn1 -- Pipe_OUT/RConn1
  2-Way Directional Valve1/RConn1 -- Hydraulic Pressure Sensor/LConn1 -- Hydraulic Pipeline/LConn1
  2-Way Directional Valve2/LConn2 -- Hydraulic Pipeline1/RConn1
  2-Way Directional Valve1/LConn2 -- pipe_IN/RConn1
  Hydraulic Pipeline/RConn1 -- Variable Head Two-Arm Tank/RConn2
  2-Way Directional Valve2/LConn1 -- Valve Control2/LConn1
  Valve Control1/LConn1 -- 2-Way Directional Valve1/LConn1
  Hydraulic Reference/LConn1 -- Hydraulic Pressure Sensor/RConn1
  PS-Simulink Converter1/LConn1 -- Hydraulic Pressure Sensor/RConn2
  Hydraulic Reference1/LConn1 -- Hydraulic Pressure Sensor1/RConn1
  PS-Simulink Converter2/LConn1 -- Hydraulic Pressure Sensor1/RConn2

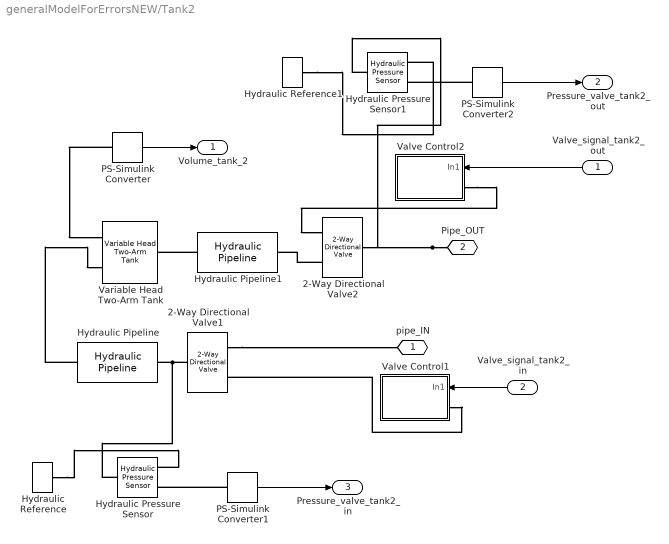
== system generalModelForErrorsNEW/Tank2 ==
  Valve_signal_tank2_out : Inport
  Valve_signal_tank2_in : Inport  Port=2
  2-Way Directional Valve1 : sh_lib/Valves/Directional Valves/2-Way Directional Valve  mdl_type=1  area_max=passage_max_area m^2  opening_max=valve_stroke m  opening_tab=[ -0.002 0 0.002 0.005 0.015 ] m  area_tab=[ 1e-9 2.0352e-7 4.0736e-5 1.1438e-4 3.4356e-4 ] m^2  pressure_tab=[ -1e+7 -5e+6 -2e+6 2e+6 5e+6 1e+7 ] Pa  flow_rate_tab=[ -1e-7 -7.0711e-8 -4.4721e-8 4.4721e-8 7.0711e-8 1e-7; -2.0352e-5 -1.4391e-5 -9.1017e-6 9.1017e-6 1.4391e-5 2.0352e-5; -0.0040736 -0.0028805 -0.0018218 0.0018218 0.0028805 0.0040736; -0.011438 -0.0080879 -0.0051152 0.0051152 0.0080879 0.011438; -0.034356 -0.024293 -0.015364 0.015364 0.024293 0.034356 ] m^3/s  interp_method=1  extrap_method=1  C_d=0.7  x_0=valve_stroke m  Re_cr=12  A_leak=1e-12 m^2
  2-Way Directional Valve2 : sh_lib/Valves/Directional Valves/2-Way Directional Valve  mdl_type=1  area_max=passage_max_area m^2  opening_max=valve_stroke m  opening_tab=[ -0.002 0 0.002 0.005 0.015 ] m  area_tab=[ 1e-9 2.0352e-7 4.0736e-5 1.1438e-4 3.4356e-4 ] m^2  pressure_tab=[ -1e+7 -5e+6 -2e+6 2e+6 5e+6 1e+7 ] Pa  flow_rate_tab=[ -1e-7 -7.0711e-8 -4.4721e-8 4.4721e-8 7.0711e-8 1e-7; -2.0352e-5 -1.4391e-5 -9.1017e-6 9.1017e-6 1.4391e-5 2.0352e-5; -0.0040736 -0.0028805 -0.0018218 0.0018218 0.0028805 0.0040736; -0.011438 -0.0080879 -0.0051152 0.0051152 0.0080879 0.011438; -0.034356 -0.024293 -0.015364 0.015364 0.024293 0.034356 ] m^3/s  interp_method=1  extrap_method=1  C_d=0.7  x_0=valve_stroke m  Re_cr=12  A_leak=1e-12 m^2
  Hydraulic Pipeline : sh_lib/Pipelines/Hydraulic Pipeline  cs_type=1  d_in=pipe_diameter m  area=1e-4 m^2  D_h=0.0112 m  s_factor=64  length=pipe_length_short m  length_ad=1 m  roughness=1.5e-5 m  Re_lam=2e+3  Re_turb=4e+3  wall_type=1  pr_r_coef=2e-12 m/Pa  time_const=0.01 s  k_sh=1.4  initial_pressure=initial_pressure Pa
  Hydraulic Pipeline1 : sh_lib/Pipelines/Hydraulic Pipeline  cs_type=1  d_in=pipe_diameter m  area=1e-4 m^2  D_h=0.0112 m  s_factor=64  length=pipe_length_short m  length_ad=1 m  roughness=1.5e-5 m  Re_lam=2e+3  Re_turb=4e+3  wall_type=1  pr_r_coef=2e-12 m/Pa  time_const=0.01 s  k_sh=1.4  initial_pressure=initial_pressure Pa
  Hydraulic Pressure Sensor : fl_lib/Hydraulic/Hydraulic Sensors/Hydraulic Pressure Sensor
  Hydraulic Pressure Sensor1 : fl_lib/Hydraulic/Hydraulic Sensors/Hydraulic Pressure Sensor
  Hydraulic Reference : fl_lib/Hydraulic/Hydraulic Elements/Hydraulic Reference
  Hydraulic Reference1 : fl_lib/Hydraulic/Hydraulic Elements/Hydraulic Reference
  PS-Simulink Converter : nesl_utility/PS-Simulink Converter  PhysicalDomain=network_engine_domain  SubClassName=ps_output  LeftPortType=input  RightPortType=output  PseudoPeriodic=off  Frequencies=[]  Unit=1  AffineConversion=off
  PS-Simulink Converter1 : nesl_utility/PS-Simulink Converter  PhysicalDomain=network_engine_domain  SubClassName=ps_output  LeftPortType=input  RightPortType=output  PseudoPeriodic=off  Frequencies=[]  Unit=1  AffineConversion=off
  PS-Simulink Converter2 : nesl_utility/PS-Simulink Converter  PhysicalDomain=network_engine_domain  SubClassName=ps_output  LeftPortType=input  RightPortType=output  PseudoPeriodic=off  Frequencies=[]  Unit=1  AffineConversion=off
  Valve Control1 : Subsystem
  Valve Control2 : Subsystem
  Variable Head Two-Arm Tank : sh_lib/Low-Pressure Blocks/Variable Head Two-Arm Tank  init_volume=1 m^3  press=pressurization_mini Pa  level_spec=1  tank_area=10 m^2  fluid_volume_tab=[ 0 0.0028 0.0065 0.0114 0.0176 0.0252 0.0344 0.0436 0.0512 0.0574 0.0623 0.066 0.0688 0.0707 0.07199999999999999 0.0727 ] m^3  fluid_level_tab=[ 0 0.02 0.04 0.06 0.08 0.1 0.12 0.14 0.16 0.18 0.2 0.22 0.24 0.26 0.28 0.3 ] m  pipe_diam_A=pipe_diameter m  loss_coeff_A=1.2  pipe_diam_B=pipe_diameter m  height_B=portb_height m  loss_coeff_B=1.2  interp_method=1  extrap_method=1
  pipe_IN : PMIOPort  Port=1  Side=Left
  Pipe_OUT : PMIOPort  Port=2  Side=Right
  Volume_tank_2 : Outport
  Pressure_valve_tank2_out : Outport  Port=2
  Pressure_valve_tank2_in : Outport  Port=3
  wires:
  PS-Simulink Converter/1 -> Volume_tank_2/1
  Valve_signal_tank2_out/1 -> Valve Control2/1(In1)
  Valve_signal_tank2_in/1 -> Valve Control1/1(In1)
  PS-Simulink Converter1/1 -> Pressure_valve_tank2_in/1
  PS-Simulink Converter2/1 -> Pressure_valve_tank2_out/1
  connections:
  Hydraulic Pipeline1/LConn1 -- Variable Head Two-Arm Tank/LConn1
  PS-Simulink Converter/LConn1 -- Variable Head Two-Arm Tank/RConn1
  Pipe_OUT/RConn1 -- Hydraulic Pressure Sensor1/LConn1 -- 2-Way Directional Valve2/RConn1
  Hydraulic Pipeline/LConn1 -- Hydraulic Pressure Sensor/LConn1 -- 2-Way Directional Valve1/RConn1
  2-Way Directional Valve2/LConn2 -- Hydraulic Pipeline1/RConn1
  2-Way Directional Valve1/LConn2 -- pipe_IN/RConn1
  Hydraulic Pipeline/RConn1 -- Variable Head Two-Arm Tank/RConn2
  Valve Control2/LConn1 -- 2-Way Directional Valve2/LConn1
  Valve Control1/LConn1 -- 2-Way Directional Valve1/LConn1
  Hydraulic Reference/LConn1 -- Hydraulic Pressure Sensor/RConn1
  PS-Simulink Converter1/LConn1 -- Hydraulic Pressure Sensor/RConn2
  Hydraulic Reference1/LConn1 -- Hydraulic Pressure Sensor1/RConn1
  PS-Simulink Converter2/LConn1 -- Hydraulic Pressure Sensor1/RConn2

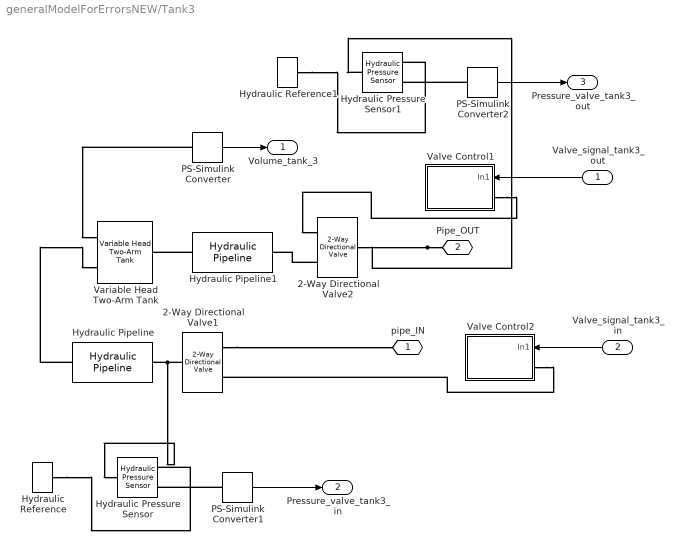
== system generalModelForErrorsNEW/Tank3 ==
  Valve_signal_tank3_out : Inport
  Valve_signal_tank3_in : Inport  Port=2
  2-Way Directional Valve1 : sh_lib/Valves/Directional Valves/2-Way Directional Valve  mdl_type=1  area_max=passage_max_area m^2  opening_max=valve_stroke m  opening_tab=[ -0.002 0 0.002 0.005 0.015 ] m  area_tab=[ 1e-9 2.0352e-7 4.0736e-5 1.1438e-4 3.4356e-4 ] m^2  pressure_tab=[ -1e+7 -5e+6 -2e+6 2e+6 5e+6 1e+7 ] Pa  flow_rate_tab=[ -1e-7 -7.0711e-8 -4.4721e-8 4.4721e-8 7.0711e-8 1e-7; -2.0352e-5 -1.4391e-5 -9.1017e-6 9.1017e-6 1.4391e-5 2.0352e-5; -0.0040736 -0.0028805 -0.0018218 0.0018218 0.0028805 0.0040736; -0.011438 -0.0080879 -0.0051152 0.0051152 0.0080879 0.011438; -0.034356 -0.024293 -0.015364 0.015364 0.024293 0.034356 ] m^3/s  interp_method=1  extrap_method=1  C_d=0.7  x_0=valve_stroke m  Re_cr=12  A_leak=1e-12 m^2
  2-Way Directional Valve2 : sh_lib/Valves/Directional Valves/2-Way Directional Valve  mdl_type=1  area_max=passage_max_area m^2  opening_max=valve_stroke m  opening_tab=[ -0.002 0 0.002 0.005 0.015 ] m  area_tab=[ 1e-9 2.0352e-7 4.0736e-5 1.1438e-4 3.4356e-4 ] m^2  pressure_tab=[ -1e+7 -5e+6 -2e+6 2e+6 5e+6 1e+7 ] Pa  flow_rate_tab=[ -1e-7 -7.0711e-8 -4.4721e-8 4.4721e-8 7.0711e-8 1e-7; -2.0352e-5 -1.4391e-5 -9.1017e-6 9.1017e-6 1.4391e-5 2.0352e-5; -0.0040736 -0.0028805 -0.0018218 0.0018218 0.0028805 0.0040736; -0.011438 -0.0080879 -0.0051152 0.0051152 0.0080879 0.011438; -0.034356 -0.024293 -0.015364 0.015364 0.024293 0.034356 ] m^3/s  interp_method=1  extrap_method=1  C_d=0.7  x_0=valve_stroke m  Re_cr=12  A_leak=1e-12 m^2
  Hydraulic Pipeline : sh_lib/Pipelines/Hydraulic Pipeline  cs_type=1  d_in=pipe_diameter m  area=1e-4 m^2  D_h=0.0112 m  s_factor=64  length=pipe_length_short m  length_ad=1 m  roughness=1.5e-5 m  Re_lam=2e+3  Re_turb=4e+3  wall_type=1  pr_r_coef=2e-12 m/Pa  time_const=0.01 s  k_sh=1.4  initial_pressure=initial_pressure Pa
  Hydraulic Pipeline1 : sh_lib/Pipelines/Hydraulic Pipeline  cs_type=1  d_in=pipe_diameter m  area=1e-4 m^2  D_h=0.0112 m  s_factor=64  length=pipe_length_short m  length_ad=1 m  roughness=1.5e-5 m  Re_lam=2e+3  Re_turb=4e+3  wall_type=1  pr_r_coef=2e-12 m/Pa  time_const=0.01 s  k_sh=1.4  initial_pressure=initial_pressure Pa
  Hydraulic Pressure Sensor : fl_lib/Hydraulic/Hydraulic Sensors/Hydraulic Pressure Sensor
  Hydraulic Pressure Sensor1 : fl_lib/Hydraulic/Hydraulic Sensors/Hydraulic Pressure Sensor
  Hydraulic Reference : fl_lib/Hydraulic/Hydraulic Elements/Hydraulic Reference
  Hydraulic Reference1 : fl_lib/Hydraulic/Hydraulic Elements/Hydraulic Reference
  PS-Simulink Converter : nesl_utility/PS-Simulink Converter  PhysicalDomain=network_engine_domain  SubClassName=ps_output  LeftPortType=input  RightPortType=output  PseudoPeriodic=off  Frequencies=[]  Unit=1  AffineConversion=off
  PS-Simulink Converter1 : nesl_utility/PS-Simulink Converter  PhysicalDomain=network_engine_domain  SubClassName=ps_output  LeftPortType=input  RightPortType=output  PseudoPeriodic=off  Frequencies=[]  Unit=1  AffineConversion=off
  PS-Simulink Converter2 : nesl_utility/PS-Simulink Converter  PhysicalDomain=network_engine_domain  SubClassName=ps_output  LeftPortType=input  RightPortType=output  PseudoPeriodic=off  Frequencies=[]  Unit=1  AffineConversion=off
  Valve Control1 : Subsystem
  Valve Control2 : Subsystem
  Variable Head Two-Arm Tank : sh_lib/Low-Pressure Blocks/Variable Head Two-Arm Tank  init_volume=1 m^3  press=pressurization_mini Pa  level_spec=1  tank_area=10 m^2  fluid_volume_tab=[ 0 0.0028 0.0065 0.0114 0.0176 0.0252 0.0344 0.0436 0.0512 0.0574 0.0623 0.066 0.0688 0.0707 0.07199999999999999 0.0727 ] m^3  fluid_level_tab=[ 0 0.02 0.04 0.06 0.08 0.1 0.12 0.14 0.16 0.18 0.2 0.22 0.24 0.26 0.28 0.3 ] m  pipe_diam_A=pipe_diameter m  loss_coeff_A=1.2  pipe_diam_B=pipe_diameter m  height_B=portb_height m  loss_coeff_B=1.2  interp_method=1  extrap_method=1
  pipe_IN : PMIOPort  Port=1  Side=Left
  Pipe_OUT : PMIOPort  Port=2  Side=Right
  Volume_tank_3 : Outport
  Pressure_valve_tank3_in : Outport  Port=2
  Pressure_valve_tank3_out : Outport  Port=3
  wires:
  PS-Simulink Converter/1 -> Volume_tank_3/1
  PS-Simulink Converter1/1 -> Pressure_valve_tank3_in/1
  PS-Simulink Converter2/1 -> Pressure_valve_tank3_out/1
  Valve_signal_tank3_out/1 -> Valve Control1/1(In1)
  Valve_signal_tank3_in/1 -> Valve Control2/1(In1)
  connections:
  Hydraulic Pipeline1/LConn1 -- Variable Head Two-Arm Tank/LConn1
  PS-Simulink Converter/LConn1 -- Variable Head Two-Arm Tank/RConn1
  Pipe_OUT/RConn1 -- Hydraulic Pressure Sensor1/LConn1 -- 2-Way Directional Valve2/RConn1
  Hydraulic Pipeline/LConn1 -- Hydraulic Pressure Sensor/LConn1 -- 2-Way Directional Valve1/RConn1
  2-Way Directional Valve2/LConn2 -- Hydraulic Pipeline1/RConn1
  2-Way Directional Valve1/LConn2 -- pipe_IN/RConn1
  Hydraulic Pipeline/RConn1 -- Variable Head Two-Arm Tank/RConn2
  Valve Control1/LConn1 -- 2-Way Directional Valve2/LConn1
  Valve Control2/LConn1 -- 2-Way Directional Valve1/LConn1
  Hydraulic Reference/LConn1 -- Hydraulic Pressure Sensor/RConn1
  PS-Simulink Converter1/LConn1 -- Hydraulic Pressure Sensor/RConn2
  Hydraulic Reference1/LConn1 -- Hydraulic Pressure Sensor1/RConn1
  PS-Simulink Converter2/LConn1 -- Hydraulic Pressure Sensor1/RConn2

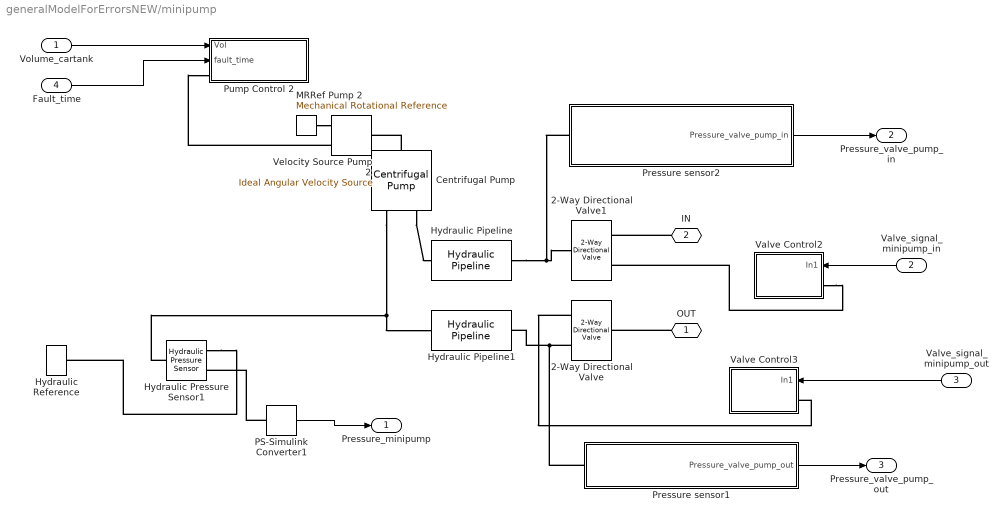
== system generalModelForErrorsNEW/minipump ==
  Volume_cartank : Inport
  Valve_signal_minipump_in : Inport  Port=2
  Valve_signal_minipump_out : Inport  Port=3
  Fault_time : Inport  Port=4
  2-Way Directional Valve : sh_lib/Valves/Directional Valves/2-Way Directional Valve  mdl_type=1  area_max=passage_max_area m^2  opening_max=valve_stroke m  opening_tab=[ -0.002 0 0.002 0.005 0.015 ] m  area_tab=[ 1e-9 2.0352e-7 4.0736e-5 1.1438e-4 3.4356e-4 ] m^2  pressure_tab=[ -1e+7 -5e+6 -2e+6 2e+6 5e+6 1e+7 ] Pa  flow_rate_tab=[ -1e-7 -7.0711e-8 -4.4721e-8 4.4721e-8 7.0711e-8 1e-7; -2.0352e-5 -1.4391e-5 -9.1017e-6 9.1017e-6 1.4391e-5 2.0352e-5; -0.0040736 -0.0028805 -0.0018218 0.0018218 0.0028805 0.0040736; -0.011438 -0.0080879 -0.0051152 0.0051152 0.0080879 0.011438; -0.034356 -0.024293 -0.015364 0.015364 0.024293 0.034356 ] m^3/s  interp_method=1  extrap_method=1  C_d=0.7  x_0=valve_stroke m  Re_cr=12  A_leak=1e-12 m^2
  2-Way Directional Valve1 : sh_lib/Valves/Directional Valves/2-Way Directional Valve  mdl_type=1  area_max=passage_max_area m^2  opening_max=valve_stroke m  opening_tab=[ -0.002 0 0.002 0.005 0.015 ] m  area_tab=[ 1e-9 2.0352e-7 4.0736e-5 1.1438e-4 3.4356e-4 ] m^2  pressure_tab=[ -1e+7 -5e+6 -2e+6 2e+6 5e+6 1e+7 ] Pa  flow_rate_tab=[ -1e-7 -7.0711e-8 -4.4721e-8 4.4721e-8 7.0711e-8 1e-7; -2.0352e-5 -1.4391e-5 -9.1017e-6 9.1017e-6 1.4391e-5 2.0352e-5; -0.0040736 -0.0028805 -0.0018218 0.0018218 0.0028805 0.0040736; -0.011438 -0.0080879 -0.0051152 0.0051152 0.0080879 0.011438; -0.034356 -0.024293 -0.015364 0.015364 0.024293 0.034356 ] m^3/s  interp_method=1  extrap_method=1  C_d=0.7  x_0=valve_stroke m  Re_cr=12  A_leak=1e-12 m^2
  Centrifugal Pump : sh_lib/Pumps and Motors/Centrifugal Pump  mdl_type=1  c_1=326.8 Pa/(kg/m^3)  c_2=3.104e+4 Pa*s/kg  c_3=1.097e+7 Pa*s^2/(kg*m^3)  c_4=2.136e+5 Pa*s^2/(kg*m^3)  c_f=0.8  design_del=130 lpm  ref_velocity=1.77e+3 rpm  ref_density=920 kg/m^3  leak_resistance=1e+8 Pa/(m^3/s)  T_const=0.1 N*m  trq_press_coeff=1e-6 N*m/Pa  pump_del_1D=[ 0 28 90 130 154 182 ] lpm  press_diff_1D=[ 2.6 2.4 2 1.6 1.2 0.8 ] bar  pump_del_power_1D=[ 0 20 40 60 80 100 120 140 160 ] lpm  power_1D=[ 220 280 310 360 390 420 480 500 550 ] W  pump_del_2D=[ 0 50 100 150 200 250 300 350 ] lpm  pump_vel_2D=[ 3.2e+3 3.3e+3 3.4e+3 3.5e+3 ] rpm  press_diff_2D=[ 8.300000000000001 8.800000000000001 9.300000000000001 9.9; 7.8 8.300000000000001 8.800000000000001 9.4; 7.2 7.6 8.199999999999999 8.699999999999999; 6.5 7 7.5 8; 5.6 6.1 6.6 7.1; 4.7 5.2 5.7 6.2; 3.4 4 4.4 4.9; 2.3 2.7 3.4 3.6 ] bar  pump_del_power_2D=[ 0 50 100 150 200 250 300 350 ] lpm  power_2D=[ 1.223e+3 1.341e+3 1.467e+3 1.6e+3; 1.414e+3 1.551e+3 1.696e+3 1.85e+3; 1.636e+3 1.794e+3 1.962e+3 2.14e+3; 1.941e+3 2.129e+3 2.326e+3 2.54e+3; 2.224e+3 2.439e+3 2.66e+3 2.91e+3; 2.453e+3 2.691e+3 2.947e+3 3.21e+3; 2.757e+3 3.024e+3 3.307e+3 3.608e+3; 2.945e+3 3.23e+3 3.533e+3 3.854e+3 ] W  interp_method=1  extrap_method=1
  Hydraulic Pipeline : sh_lib/Pipelines/Hydraulic Pipeline  cs_type=1  d_in=pipe_diameter m  area=1e-4 m^2  D_h=0.0112 m  s_factor=64  length=pipe_length_short m  length_ad=1 m  roughness=1.5e-5 m  Re_lam=2e+3  Re_turb=4e+3  wall_type=1  pr_r_coef=2e-12 m/Pa  time_const=0.01 s  k_sh=1.4  initial_pressure=initial_pressure Pa
  Hydraulic Pipeline1 : sh_lib/Pipelines/Hydraulic Pipeline  cs_type=1  d_in=pipe_diameter m  area=1e-4 m^2  D_h=0.0112 m  s_factor=64  length=pipe_length_short m  length_ad=1 m  roughness=1.5e-5 m  Re_lam=2e+3  Re_turb=4e+3  wall_type=1  pr_r_coef=2e-12 m/Pa  time_const=0.01 s  k_sh=1.4  initial_pressure=initial_pressure Pa
  Hydraulic Pressure Sensor1 : fl_lib/Hydraulic/Hydraulic Sensors/Hydraulic Pressure Sensor
  Hydraulic Reference : fl_lib/Hydraulic/Hydraulic Elements/Hydraulic Reference
  MRRef Pump 2 : fl_lib/Mechanical/Rotational Elements/Mechanical Rotational Reference
  PS-Simulink Converter1 : nesl_utility/PS-Simulink Converter  PhysicalDomain=network_engine_domain  SubClassName=ps_output  LeftPortType=input  RightPortType=output  PseudoPeriodic=off  Frequencies=[]  Unit=1  AffineConversion=off
  Pressure sensor1 : Subsystem
  Pressure sensor2 : Subsystem
  Pump Control 2 : Subsystem
  Valve Control2 : Subsystem
  Valve Control3 : Subsystem
  Velocity Source Pump 2 : fl_lib/Mechanical/Mechanical Sources/Ideal Angular Velocity Source
  OUT : PMIOPort  Port=1  Side=Left
  IN : PMIOPort  Port=2  Side=Right
  Pressure_minipump : Outport
  Pressure_valve_pump_in : Outport  Port=2
  Pressure_valve_pump_out : Outport  Port=3
  wires:
  Volume_cartank/1 -> Pump Control 2/1(Vol)
  PS-Simulink Converter1/1 -> Pressure_minipump/1
  Valve_signal_minipump_in/1 -> Valve Control2/1(In1)
  Fault_time/1 -> Pump Control 2/2(fault_time)
  Pressure sensor2/1(Pressure_valve_pump_in) -> Pressure_valve_pump_in/1
  Pressure sensor1/1(Pressure_valve_pump_out) -> Pressure_valve_pump_out/1
  Valve_signal_minipump_out/1 -> Valve Control3/1(In1)
  connections:
  Hydraulic Pipeline/LConn1 -- Pressure sensor2/LConn1 -- 2-Way Directional Valve1/RConn1
  Centrifugal Pump/RConn2 -- Hydraulic Pipeline/RConn1
  2-Way Directional Valve/LConn2 -- Pressure sensor1/LConn1 -- Hydraulic Pipeline1/RConn1
  IN/RConn1 -- 2-Way Directional Valve1/LConn2
  OUT/RConn1 -- 2-Way Directional Valve/RConn1
  MRRef Pump 2/LConn1 -- Velocity Source Pump 2/RConn2
  Centrifugal Pump/LConn1 -- Velocity Source Pump 2/LConn1
  Centrifugal Pump/RConn1 -- Hydraulic Pressure Sensor1/LConn1 -- Hydraulic Pipeline1/LConn1
  Velocity Source Pump 2/RConn1 -- Pump Control 2/LConn1
  PS-Simulink Converter1/LConn1 -- Hydraulic Pressure Sensor1/RConn2
  Valve Control2/LConn1 -- 2-Way Directional Valve1/LConn1
  2-Way Directional Valve/LConn1 -- Valve Control3/LConn1
  Hydraulic Pressure Sensor1/RConn1 -- Hydraulic Reference/LConn1

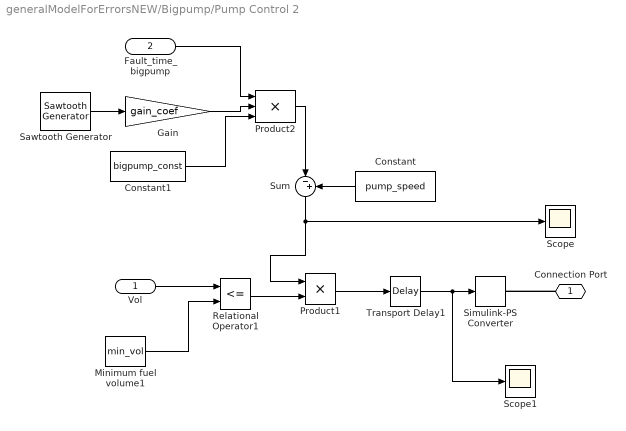
== system generalModelForErrorsNEW/Bigpump/Pump Control 2 ==
  Vol : Inport
  Fault_time_bigpump : Inport  Port=2
  Constant : Constant  Value=pump_speed
  Constant1 : Constant  Value=bigpump_const
  Gain : Gain  Gain=gain_coef
  Minimum fuel volume1 : Constant  Value=min_vol
  Product1 : Product  RndMeth=Zero
  Product2 : Product  Inputs=3
  Relational Operator1 : RelationalOperator  Operator=<=  OutDataTypeStr=boolean  RndMeth=Nearest
  Sawtooth Generator : powerlib_meascontrol/Pulse & Signal Generators/Sawtooth Generator  Freq=0.0001  Phase=180  Ts=0
  Scope : Scope
  Scope1 : Scope
  Simulink-PS Converter : nesl_utility/Simulink-PS Converter  PhysicalDomain=network_engine_domain  SubClassName=ps_input  LeftPortType=input  RightPortType=output  PseudoPeriodic=off  Frequencies=[]  NoiseDistribution=none  NoiseParameters=[]  Unit=1  AffineConversion=off  InputFiltering=off  SimscapeFilterOrder=1  InputFilterTimeConstant=0.001  UdotUserProvided=1
  Sum : Sum  Inputs=|-+
  Transport Delay1 : TransportDelay  DelayTime=3
  Connection Port : PMIOPort  Port=1  Side=Left
  wires:
  Sawtooth Generator/1 -> Gain/1
  Transport Delay1/1 -> Scope1/1, Simulink-PS Converter/1
  Minimum fuel volume1/1 -> Relational Operator1/2
  Vol/1 -> Relational Operator1/1
  Relational Operator1/1 -> Product1/2
  Product1/1 -> Transport Delay1/1
  Constant/1 -> Sum/2
  Sum/1 -> Product1/1, Scope/1
  Fault_time_bigpump/1 -> Product2/1
  Gain/1 -> Product2/2
  Product2/1 -> Sum/1
  Constant1/1 -> Product2/3
  connections:
  Connection Port/RConn1 -- Simulink-PS Converter/RConn1

== system generalModelForErrorsNEW/Bigpump/Valve Control2 ==
  In1 : Inport
  Constant : Constant  Value=ws_sample_time_end_valve_bigpump_in
  Logical Operator : Logic  AllPortsSameDT=off  OutDataTypeStr=boolean
  Product : Product
  S2PS1 : nesl_utility/Simulink-PS Converter  PhysicalDomain=network_engine_domain  SubClassName=ps_input  LeftPortType=input  RightPortType=output  PseudoPeriodic=off  Frequencies=[]  NoiseDistribution=none  NoiseParameters=[]  Unit=1  AffineConversion=off  InputFiltering=off  SimscapeFilterOrder=1  InputFilterTimeConstant=.001  UdotUserProvided=0
  Signal Builder : Subsystem  Tag=STV Subsys  LoadFcn=sigbuilder_block('load');  StartFcn=sigbuilder_block('start');  StopFcn=sigbuilder_block('stop');  ClipboardFcn=sigbuilder_block('clipboard');  mask(Sigbuilder block){tuvar=[0:10]}
      mask help: Simulink:masks:SigbuilderBlock_MD
      mask init:
      | if ~strcmp(get_param(bdroot(gcbh),'SimulationStatus'),'stopped') tuvar = sigbuilder_block('maskInit'); end
      settings: CopyFcn=sigbuilder_block('copy');  DeleteFcn=sigbuilder_block('delete');  ModelCloseFcn=sigbuilder_block('modelClose');  PreSaveFcn=sigbuilder_block('preSave');  PauseFcn=sigbuilder_block('pause');  ContinueFcn=sigbuilder_block('continue');  NameChangeFcn=sigbuilder_block('namechange');  OpenFcn=sigbuilder_block('open',[1024.5 -234 1440 722.25 ]);  CloseFcn=sigbuilder_block('close');
      mask Display: plot(0, 0, 100, 100,[2, 2, 32, 32, 2], [68, 8, 8, 68, 68],[32, 2], [38, 38], [32, 19, 2],[53, 60, 44], [32, 17, 17, 2],[16, 16, 31, 31]);txt = getActiveGroup(gcbh);text(2, 100, txt,'verticalAlignment', 'top');
  Transport Delay : TransportDelay  DelayTime=ws_fault_time
  Valve Actuator : sh_lib/Valves/Valve Actuators/Valve Actuator  valve_stroke=valve_stroke m  time_constant=0.01 s  gain=valve_gain*5 m
  Signal : PMIOPort  Port=1  Side=Left
  wires:
  Product/1 -> S2PS1/1
  In1/1 -> Logical Operator/1
  Signal Builder/1(Signal 2) -> Transport Delay/1
  Transport Delay/1 -> Product/2
  Constant/1 -> Logical Operator/2
  Logical Operator/1 -> Product/1
  connections:
  Valve Actuator/RConn1 -- Signal/RConn1
  Valve Actuator/LConn1 -- S2PS1/RConn1
